simulink model "S_linkreach_target_control"  (R2025b)
settings: Solver=VariableStepAuto  StartTime=0.0  StopTime=10.0  RelTol=1e-3
settings Model: Creator=Wing  LastModifiedBy=allen

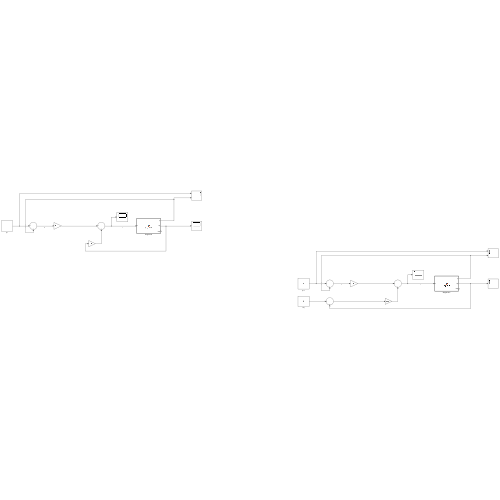
[thumbnail: Simulink's stored preview of the top-level diagram]
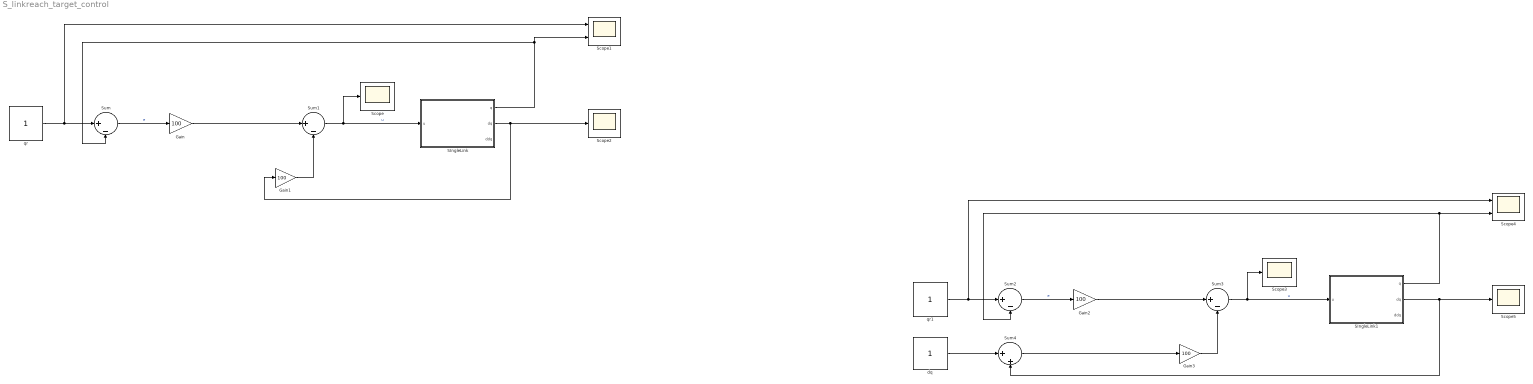
== system S_linkreach_target_control ==
  Gain{,1..3} (4 alike) : Gain  Gain=100
  SIngleLink : MATLAB Function  TreatAsAtomicUnit=on
  SIngleLink1 : MATLAB Function  TreatAsAtomicUnit=on
  Scope{,2..3,5} (4 alike) : Scope
      Scope2 settings: DataLoggingVariableName=ScopeData2
      Scope3 settings: DataLoggingVariableName=ScopeData3
      Scope5 settings: DataLoggingVariableName=ScopeData5
  Scope1 : Scope  NumInputPorts=2
  Scope4 : Scope  NumInputPorts=2
      settings: DataLoggingVariableName=ScopeData4
  Sum{,1..3} (4 alike) : Sum  Inputs=|+-
  Sum4 : Sum  Inputs=|++
  dq : Constant
  qr : Constant
  qr1 : Constant
  wires:
  qr/1 -> Sum/1, Scope1/1
  Sum/1 -> Gain/1  "e"
  Gain/1 -> Sum1/1
  Gain1/1 -> Sum1/2
  Sum1/1 -> SIngleLink/1(u), Scope/1  "u"
  SIngleLink/1(q) -> Scope1/2, Sum/2
  SIngleLink/2(dq) -> Scope2/1, Gain1/1
  Gain2/1 -> Sum3/1
  Sum3/1 -> SIngleLink1/1(u), Scope3/1  "u"
  qr1/1 -> Sum2/1, Scope4/1
  Gain3/1 -> Sum3/2
  SIngleLink1/1(q) -> Scope4/2, Sum2/2
  SIngleLink1/2(dq) -> Sum4/2, Scope5/1
  Sum2/1 -> Gain2/1  "e"
  dq/1 -> Sum4/1
  Sum4/1 -> Gain3/1

== matlab function S_linkreach_target_control/SIngleLink ==
  data: u input; q output; dq output; ddq output
function [q, dq, ddq] = SingleLink(u)

== matlab function S_linkreach_target_control/SIngleLink1 ==
  data: u input; q output; dq output; ddq output
function [q, dq, ddq] = SingleLink(u)
